simulink model "questao2a"  (Simulink 3.00)
settings: Solver=ode45  StartTime=0.0  StopTime=3  RelTol=1e-3
libraries: simulink3 x1

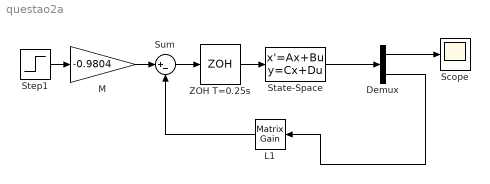
== system questao2a ==
  Demux : Demux  Outputs=2
  L1 : simulink3/Math/Matrix Gain  Orientation=left  K=[255.6418 90.8066 10.9089]
  M : Gain  Gain=-0.9804  SaturateOnIntegerOverflow=on
  Scope : Scope
      settings: TimeRange=auto  YMin=-5  YMax=5  SaveToWorkspace=off  SaveName=ScopeData
  State-Space : StateSpace  A=[0 1 0;23.75 5.25 1;-2 0 1]  B=[0;0;1]  C=[1 0 1;eye(3,3)]  D=[0;0;0;0]  X0=0
  Step1 : Step  Time=0  Before=0  After=1  SampleTime=0
  Sum : Sum  Inputs=|+-  SaturateOnIntegerOverflow=on
  ZOH T=0.25s : ZeroOrderHold  SampleTime=0.25
  wires:
  M/1 -> Sum/1
  Step1/1 -> M/1
  L1/1 -> Sum/2
  Sum/1 -> ZOH T=0.25s/1
  ZOH T=0.25s/1 -> State-Space/1
  Demux/1 -> Scope/1
  State-Space/1 -> Demux/1
  Demux/2 -> L1/1
